simulink model "a_sign"  (R2019b)
settings: Solver=VariableStepAuto  StartTime=0.0  StopTime=10.0  RelTol=1e-3
values from neighbouring files (symbols this model uses):
  Tf1 = 0.06    [rotary_ip_lq.m]
libraries: cstblocks x4
settings Model: Creator=Noritaka Okayasu  LastModifiedBy=Noritaka Okayasu

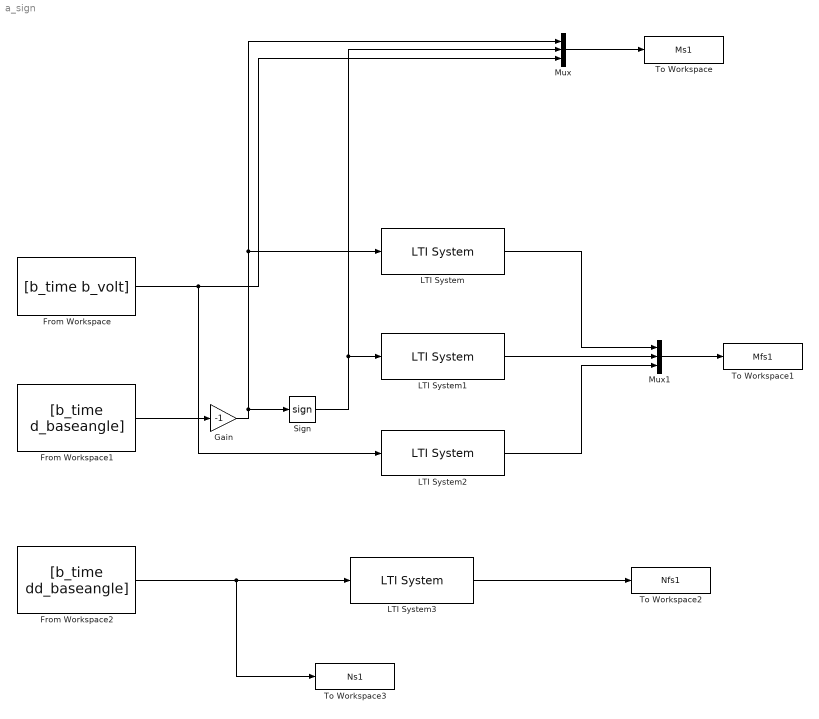
== system a_sign ==
  From Workspace : FromWorkspace  VariableName=[b_time b_volt]  SampleTime=0
  From Workspace1 : FromWorkspace  VariableName=[b_time d_baseangle]  SampleTime=0
  From Workspace2 : FromWorkspace  VariableName=[b_time dd_baseangle]  SampleTime=0
  Gain : Gain  Gain=-1
  LTI System{,1..3} (4 alike) : cstblocks/LTI System  sys=tf(1, [Tf1 1])^3  IC=[]
  Mux : Mux  Inputs=3
  Mux1 : Mux  Inputs=3
  Sign : Signum
  To Workspace : ToWorkspace  VariableName=Ms1  SampleTime=-1
  To Workspace1 : ToWorkspace  VariableName=Mfs1  SampleTime=-1
  To Workspace2 : ToWorkspace  VariableName=Nfs1  SampleTime=-1
  To Workspace3 : ToWorkspace  VariableName=Ns1  SampleTime=-1
  wires:
  From Workspace/1 -> LTI System2/1, Mux/3
  From Workspace1/1 -> Gain/1
  Gain/1 -> Sign/1, LTI System/1, Mux/1
  Sign/1 -> LTI System1/1, Mux/2
  Mux/1 -> To Workspace/1
  LTI System/1 -> Mux1/1
  LTI System1/1 -> Mux1/2
  LTI System2/1 -> Mux1/3
  From Workspace2/1 -> To Workspace3/1, LTI System3/1
  Mux1/1 -> To Workspace1/1
  LTI System3/1 -> To Workspace2/1
